simulink library "bdot_controller_lib"  (R2016b)
settings: Solver=ode45  StartTime=0.0  StopTime=10.0  RelTol=1e-3  EnableMultiTasking=on
undefined symbols (not defined in the file or in its folder): fsw_params
libraries: simulink x1
settings Model: Creator=Taylor  LastModifiedBy=Taylor
settings DataIOCC: LimitDataPoints=on
settings OptimizationCC: LifeSpan=inf
settings DebuggingCC: AllowSymbolicDim=off  SFUnexpectedBacktrackingDiag=warning  SFNoUnconditionalDefaultTransitionDiag=warning  SFExecutionAtInitializationDiag=none
settings GRTTargetCC: TargetLangStandard=C89/C90 (ANSI)  GeneratePreprocessorConditionals=Disable all
settings ConfigComp: CovMetricSettings=dw  CovHtmlReporting=on  CovSaveCumulativeToWorkspaceVar=on  CovSaveSingleToWorkspaceVar=on  CovExternalEMLEnable=off

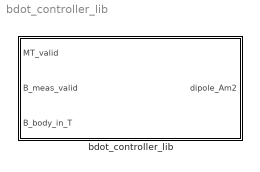
== system bdot_controller_lib ==
  bdot_controller_lib : Subsystem

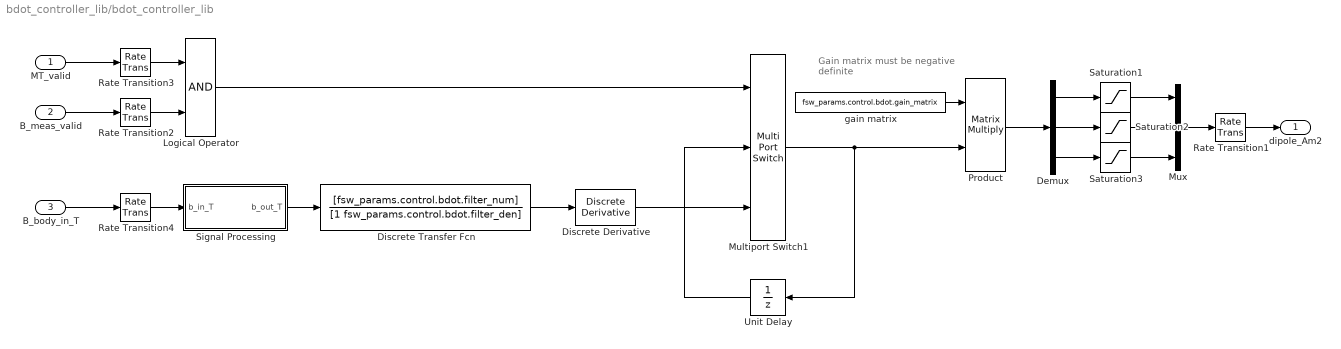
== system bdot_controller_lib/bdot_controller_lib ==
  note: Gain matrix must be
      | negative definite
  MT_valid : Inport
  B_meas_valid : Inport  Port=2
  B_body_in_T : Inport  Port=3
  Demux : Demux  Outputs=3
  Discrete Transfer Fcn : DiscreteTransferFcn  Numerator=[fsw_params.control.bdot.filter_num]  Denominator=[1 fsw_params.control.bdot.filter_den]
  Discrete Derivative : simulink/Discrete/Discrete Derivative  gainval=1.0  ICPrevScaledInput=fsw_params.control.bdot.ic.derivative  InputProcessing=Inherited  OutMin=[]  OutMax=[]  OutDataType=fixdt(1, 16)  OutScaling=2^-10  DoSatur=off
  Logical Operator : Logic  AllPortsSameDT=off  OutDataTypeStr=boolean
  Multiport Switch1 : MultiPortSwitch  DataPortOrder=Zero-based contiguous  Inputs=2
  Mux : Mux  Inputs=3
  Product : Product  Multiplication=Matrix(*)
  Rate Transition1 : RateTransition  X0=fsw_params.control.bdot.ic.RT_dig_val  OutPortSampleTimeOpt=Inherit  OutPortSampleTime=sc_params.control.sample_time_s
  Rate Transition2 : RateTransition  Deterministic=off  X0=fsw_params.control.bdot.ic.RT_b_meas_valid  OutPortSampleTime=fsw_params.control.bdot.sample_time_s
  Rate Transition3 : RateTransition  Deterministic=off  OutPortSampleTime=fsw_params.control.bdot.sample_time_s
  Rate Transition4 : RateTransition  Deterministic=off  X0=fsw_params.control.bdot.ic.RT_b_body_T  OutPortSampleTime=fsw_params.control.bdot.sample_time_s
  Saturation1 : Saturate  UpperLimit=fsw_params.actuators.magnetorquer.max_dipole_x  LowerLimit=-fsw_params.actuators.magnetorquer.max_dipole_x
  Saturation2 : Saturate  UpperLimit=fsw_params.actuators.magnetorquer.max_dipole_y  LowerLimit=-fsw_params.actuators.magnetorquer.max_dipole_y
  Saturation3 : Saturate  UpperLimit=fsw_params.actuators.magnetorquer.max_dipole_z  LowerLimit=-fsw_params.actuators.magnetorquer.max_dipole_z
  Signal Processing : Subsystem
  Unit Delay : UnitDelay  InitialCondition=fsw_params.control.bdot.ic.unit_delay  SampleTime=-1
  gain matrix : Constant  Value=fsw_params.control.bdot.gain_matrix
  dipole_Am2 : Outport
  wires:
  Saturation1/1 -> Mux/1
  Unit Delay/1 -> Multiport Switch1/2
  Rate Transition1/1 -> dipole_Am2/1
  Rate Transition4/1 -> Signal Processing/1(b_in_T)
  B_body_in_T/1 -> Rate Transition4/1
  B_meas_valid/1 -> Rate Transition2/1
  Discrete Transfer Fcn/1 -> Discrete Derivative/1
  Discrete Derivative/1 -> Multiport Switch1/3
  Signal Processing/1(b_out_T) -> Discrete Transfer Fcn/1
  Multiport Switch1/1 -> Product/2, Unit Delay/1
  gain matrix/1 -> Product/1
  Product/1 -> Demux/1
  Demux/1 -> Saturation1/1
  Demux/3 -> Saturation3/1
  Demux/2 -> Saturation2/1
  Saturation3/1 -> Mux/3
  Saturation2/1 -> Mux/2
  Mux/1 -> Rate Transition1/1
  MT_valid/1 -> Rate Transition3/1
  Rate Transition3/1 -> Logical Operator/1
  Rate Transition2/1 -> Logical Operator/2
  Logical Operator/1 -> Multiport Switch1/1

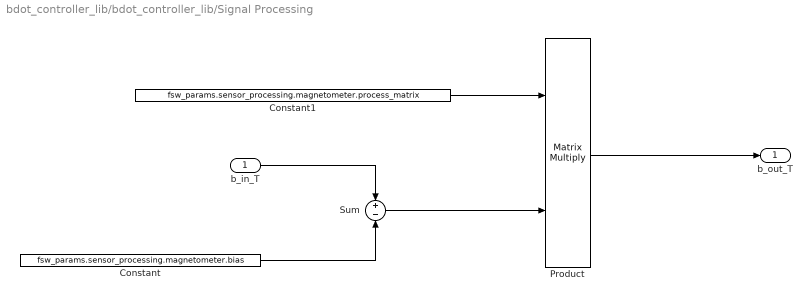
== system bdot_controller_lib/bdot_controller_lib/Signal Processing ==
  b_in_T : Inport
  Constant : Constant  Value=fsw_params.sensor_processing.magnetometer.bias  SampleTime=fsw_params.control.bdot.sample_time_s
  Constant1 : Constant  Value=fsw_params.sensor_processing.magnetometer.process_matrix  SampleTime=fsw_params.control.bdot.sample_time_s
  Product : Product  Multiplication=Matrix(*)
  Sum : Sum  Inputs=+-
  b_out_T : Outport
  wires:
  Constant/1 -> Sum/2
  b_in_T/1 -> Sum/1
  Constant1/1 -> Product/1
  Sum/1 -> Product/2
  Product/1 -> b_out_T/1
